simulink model "ZAD2_1_Model"  (R2018a)
settings: Solver=ode45  StartTime=0.0  StopTime=tend  MaxStep=Tp  RelTol=1e-3
values from neighbouring files (symbols this model uses):
  b1 = (eta1^2) *b1 + bm1 + (km1*kb1)/R1    (= 0.00702436843727)    [ZAD0_SRManCw3_Init.m]
  b2 = (eta2^2) *b2 + bm2 + (km2*kb2)/R2    (= 0.00687174794339)    [ZAD0_SRManCw3_Init.m]
  eta = diag([eta1; eta2])    [ZAD0_SRManCw3_Init.m]
  initConditionsPos = [-pi/2; 0]    [ZAD0_SRManCw3_Init.m]
  initConditionsVel = [0; 0]    [ZAD0_SRManCw3_Init.m]
  invR = inv(R)    [ZAD0_SRManCw3_Init.m]
  J1 = Jm1 + (eta1^2) * Jl1    (= 0.000358828993824)    [ZAD0_SRManCw3_Init.m]
  J2 = Jm2 + eta2^2*Jl2    (= 0.000193490125454)    [ZAD0_SRManCw3_Init.m]
  kc1 = 1 / sqrt(kd1 / ki1)    [ZAD0_SRManCw3_Init.m]
  kc2 = 1 / sqrt(kd2 / ki2)    [ZAD0_SRManCw3_Init.m]
  kd1 = omega_n1*zeta1*(2 + lambda1)*J1 - b1    (= 0.0101994232663)    [ZAD0_SRManCw3_Init.m]
  kd2 = omega_n2*zeta2*(2 + lambda2)*J2 - b2    (= 9.38965729567e-05)    [ZAD0_SRManCw3_Init.m]
  ki1 = (omega_n1^3) *lambda1*zeta1*J1    (= 0.465042375996)    [ZAD0_SRManCw3_Init.m]
  ki2 = (omega_n2^3) * lambda2*zeta2*J2    (= 0.167175468392)    [ZAD0_SRManCw3_Init.m]
  Km = diag([km1; km2])    [ZAD0_SRManCw3_Init.m]
  km1 = km    (= 0.0782)    [ZAD0_SRManCw3_Init.m]
  km2 = km    (= 0.0782)    [ZAD0_SRManCw3_Init.m]
  kp1 = (omega_n1^2) * (1 + 2*lambda1*zeta1^2)*J1    (= 0.16793196911)    [ZAD0_SRManCw3_Init.m]
  kp2 = (omega_n2^2) *(1 + 2*lambda2*zeta2^2)*J2    (= 0.0626908006471)    [ZAD0_SRManCw3_Init.m]
  omega1 = 0.6    [ZAD0_SRManCw3_Init.m]
  omega2 = 0.7    [ZAD0_SRManCw3_Init.m]
  Qd01 = 0.65    [ZAD0_SRManCw3_Init.m]
  Qd02 = 0.65    [ZAD0_SRManCw3_Init.m]
  Qd1 = 1.2    [ZAD0_SRManCw3_Init.m]
  Qd11 = 0.75    [ZAD0_SRManCw3_Init.m]
  Qd12 = 0.78    [ZAD0_SRManCw3_Init.m]
  Qd1const = 0.7    [ZAD0_SRManCw3_Init.m]
  Qd2 = 1.3    [ZAD0_SRManCw3_Init.m]
  Qd21 = 0.70    (= 0.7)    [ZAD0_SRManCw3_Init.m]
  Qd22 = 0.98    [ZAD0_SRManCw3_Init.m]
  Qd2const = 0.8    [ZAD0_SRManCw3_Init.m]
  Qd31 = 0.45    [ZAD0_SRManCw3_Init.m]
  Qd32 = 0.90    (= 0.9)    [ZAD0_SRManCw3_Init.m]
  R1 = R    (= 0.917)    [ZAD0_SRManCw3_Init.m]
  R2 = R    (= 0.917)    [ZAD0_SRManCw3_Init.m]
libraries: simulink x2
settings Model: Creator=szymon  LastModifiedBy=szymon

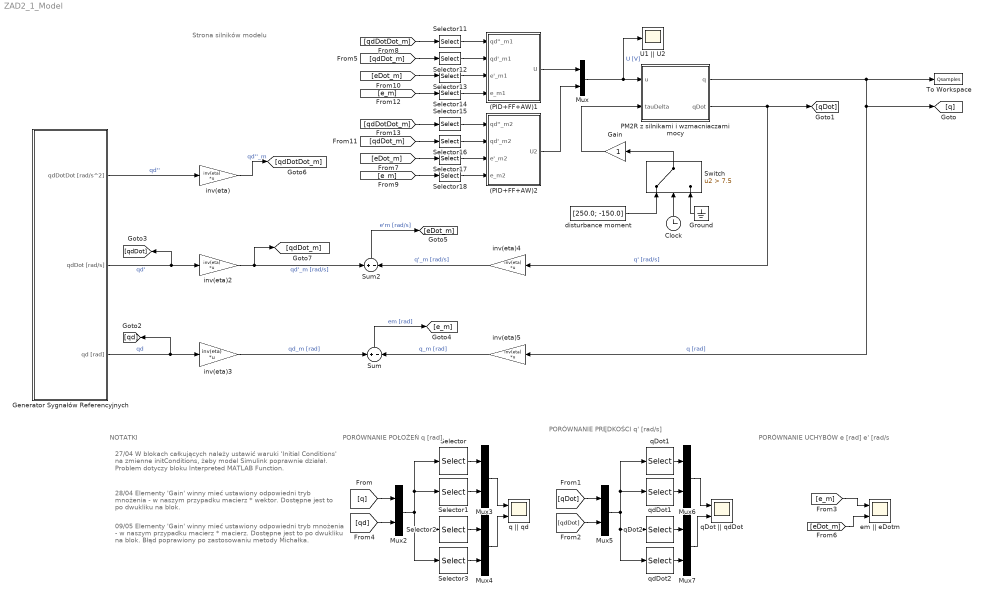
== system ZAD2_1_Model ==
  note: Strona silników modelu
  note: PORÓWNANIE POŁOŻEŃ
      | q [rad]
  note: NOTATKI
  note: 27/04 W blokach całkujących należy ustawić waruki
      | 'Initial Conditions' na zmienne initConditions, żeby model
      | Simulink poprawnie działał. Problem dotyczy bloku
      | Interpreted MATLAB Function.
  note: 28/04 Elementy 'Gain' winny mieć ustawiony odpowiedni tryb
      | mnożenia - w naszym przypadku macierz * wektor.
      | Dostępne jest to po dwukliku na blok.
  note: PORÓWNANIE PRĘDKOŚCI
      | q' [rad/s]
  note: 09/05 Elementy 'Gain' winny mieć ustawiony odpowiedni tryb
      | mnożenia - w naszym przypadku macierz * macierz.
      | Dostępne jest to po dwukliku na blok. Błąd poprawiony po
      | zastosowaniu metody Michałka.
  note: PORÓWNANIE UCHYBÓW
      | e  [rad]
      | e' [rad/s
  (PID+FF+AW)1 : Subsystem
  (PID+FF+AW)2 : Subsystem
  Clock : Clock
  Gain : Gain
  Generator Sygnałów Referencyjnych : Subsystem
  Ground : Ground
  Mux{,2..7} (7 alike) : Mux  Inputs=2
  PM2R z silnikami i wzmacniaczami mocy : Subsystem
  Selector : Selector  InputPortWidth=4  IndexOptions=Index vector (dialog)  Indices=[1]  OutputSizes=1
  Selector1 : Selector  InputPortWidth=4  IndexOptions=Index vector (dialog)  Indices=[3]  OutputSizes=1
  Selector{11..14} (4 alike) : Selector  InputPortWidth=2  IndexOptions=Index vector (dialog)  Indices=[1]  OutputSizes=1
  Selector{15..18} (4 alike) : Selector  InputPortWidth=2  IndexOptions=Index vector (dialog)  Indices=[2]  OutputSizes=1
  Selector2 : Selector  InputPortWidth=4  IndexOptions=Index vector (dialog)  Indices=[2]  OutputSizes=1
  Selector3 : Selector  InputPortWidth=4  IndexOptions=Index vector (dialog)  Indices=[4]  OutputSizes=1
  Sum : Sum  Inputs=+-
  Sum2 : Sum  Inputs=+-
  Switch : Switch  Criteria=u2 > Threshold  Threshold=7.5
  To Workspace : ToWorkspace  VariableName=Qsamples  SampleTime=-1
  U1 || U2 : Scope
  disturbance moment : Constant  Value=[250.0; -150.0]
  em || eDotm : Scope  NumInputPorts=2
  inv(eta){,2..5} (5 alike) : Gain  Gain=inv(eta)  Multiplication=Matrix(K*u)
  q || qd : Scope  NumInputPorts=2
  qDot || qdDot : Scope  NumInputPorts=2
  qDot1 : Selector  InputPortWidth=4  IndexOptions=Index vector (dialog)  Indices=[1]  OutputSizes=1
  qDot2 : Selector  InputPortWidth=4  IndexOptions=Index vector (dialog)  Indices=[2]  OutputSizes=1
  qdDot1 : Selector  InputPortWidth=4  IndexOptions=Index vector (dialog)  Indices=[3]  OutputSizes=1
  qdDot2 : Selector  InputPortWidth=4  IndexOptions=Index vector (dialog)  Indices=[4]  OutputSizes=1
  wires:
  PM2R z silnikami i wzmacniaczami mocy/2(qDot) -> inv(eta)4/1, [qDot]  "q' [rad/s]"
  PM2R z silnikami i wzmacniaczami mocy/1(q) -> inv(eta)5/1, [q], To Workspace/1  "q [rad]"
  [q] -> Mux2/1
  [qd] -> Mux2/2
  Selector/1 -> Mux3/1
  Selector1/1 -> Mux3/2
  Selector2/1 -> Mux4/1
  Selector3/1 -> Mux4/2
  Mux2/1 -> Selector3/1, Selector2/1, Selector1/1, Selector/1
  Mux3/1 -> q || qd/1
  Mux4/1 -> q || qd/2
  qDot2/1 -> Mux7/1
  Mux6/1 -> qDot || qdDot/1
  Mux7/1 -> qDot || qdDot/2
  qdDot2/1 -> Mux7/2
  [qDot] -> Mux5/1
  qdDot1/1 -> Mux6/2
  [qdDot] -> Mux5/2
  qDot1/1 -> Mux6/1
  Mux5/1 -> qdDot2/1, qDot2/1, qdDot1/1, qDot1/1
  Generator Sygnałów Referencyjnych/2(qdDot [rad/s]) -> [qdDot], inv(eta)2/1  "qd'"
  Generator Sygnałów Referencyjnych/1(qdDotDot [rad/s^2]) -> inv(eta)/1  "qd''"
  inv(eta)2/1 -> [qdDot_m], Sum2/1  "qd'_m [rad/s]"
  Mux/1 -> U1 || U2/1, PM2R z silnikami i wzmacniaczami mocy/1(u)  "U [V]"
  Sum2/1 -> [eDot_m]  "e'm [rad/s]"
  Sum/1 -> [e_m]  "em [rad]"
  Selector11/1 -> (PID+FF+AW)1/1(qd''_m1)
  Selector12/1 -> (PID+FF+AW)1/2(qd'_m1)
  Selector13/1 -> (PID+FF+AW)1/3(e'_m1)
  Selector14/1 -> (PID+FF+AW)1/4(e_m1)
  Selector15/1 -> (PID+FF+AW)2/1(qd''_m2)
  Selector16/1 -> (PID+FF+AW)2/2(qd'_m2)
  Selector17/1 -> (PID+FF+AW)2/3(e'_m2)
  Selector18/1 -> (PID+FF+AW)2/4(e_m2)
  (PID+FF+AW)1/1(U) -> Mux/1
  [e_m] -> em || eDotm/1
  inv(eta)4/1 -> Sum2/2  "q'_m [rad/s]"
  inv(eta)5/1 -> Sum/2  "q_m [rad]"
  (PID+FF+AW)2/1(U2) -> Mux/2
  [qdDot_m] -> Selector12/1
  inv(eta)/1 -> [qdDotDot_m]  "qd''_m"
  [qdDotDot_m] -> Selector11/1
  [eDot_m] -> Selector13/1
  [e_m] -> Selector14/1
  [eDot_m] -> Selector17/1
  [qdDot_m] -> Selector16/1
  [e_m] -> Selector18/1
  [qdDotDot_m] -> Selector15/1
  inv(eta)3/1 -> Sum/1  "qd_m [rad]"
  Generator Sygnałów Referencyjnych/3(qd [rad]) -> [qd], inv(eta)3/1  "qd"
  [eDot_m] -> em || eDotm/2
  Switch/1 -> Gain/1
  Ground/1 -> Switch/3
  Clock/1 -> Switch/2
  disturbance moment/1 -> Switch/1
  Gain/1 -> PM2R z silnikami i wzmacniaczami mocy/2(tauDelta)

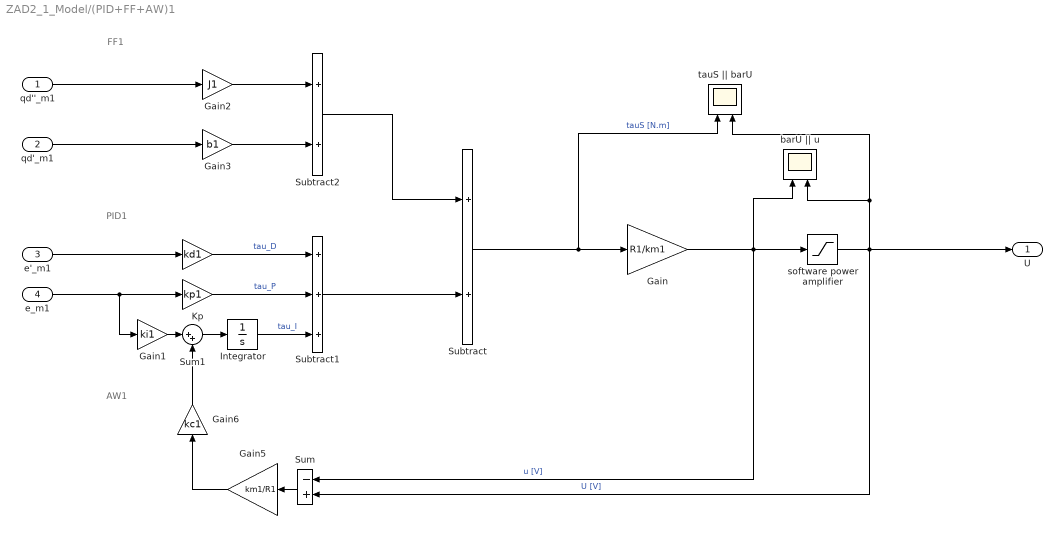
== system ZAD2_1_Model/(PID+FF+AW)1 ==
  note: AW1
  note: FF1
  note: PID1
  qd''_m1 : Inport
  qd'_m1 : Inport  Port=2
  e'_m1 : Inport  Port=3
  e_m1 : Inport  Port=4
  " " : Gain  Gain=kd1
  Gain : Gain  Gain=R1/km1
  Gain1 : Gain  Gain=ki1
  Gain2 : Gain  Gain=J1
  Gain3 : Gain  Gain=b1
  Gain5 : Gain  Gain=km1/R1
  Gain6 : Gain  Gain=kc1
  Integrator : Integrator
  Kp : Gain  Gain=kp1
  Subtract : Sum
  Subtract1 : Sum  Inputs=+++
  Subtract2 : Sum
  Sum : Sum  Inputs=-+
  Sum1 : Sum  Inputs=|++
  barU || u : Scope  NumInputPorts=2
  software power amplifier : Saturate  UpperLimit=24.0  LowerLimit=-24.0
  tauS || barU : Scope  NumInputPorts=2
  U : Outport
  wires:
  Subtract1/1 -> Subtract/2
  Subtract2/1 -> Subtract/1
  Subtract/1 -> Gain/1, tauS || barU/1  "tauS [N.m]"
  software power amplifier/1 -> U/1, tauS || barU/2, barU || u/2, Sum/2  "U [V]"
  e'_m1/1 -> " "/1
  " "/1 -> Subtract1/1  "tau_D"
  Kp/1 -> Subtract1/2  "tau_P"
  qd'_m1/1 -> Gain3/1
  Gain3/1 -> Subtract2/2
  Gain2/1 -> Subtract2/1
  qd''_m1/1 -> Gain2/1
  Gain6/1 -> Sum1/2
  Gain/1 -> Sum/1, software power amplifier/1, barU || u/1  "u [V]"
  Sum/1 -> Gain5/1
  Gain5/1 -> Gain6/1
  e_m1/1 -> Gain1/1, Kp/1
  Integrator/1 -> Subtract1/3  "tau_I"
  Gain1/1 -> Sum1/1
  Sum1/1 -> Integrator/1

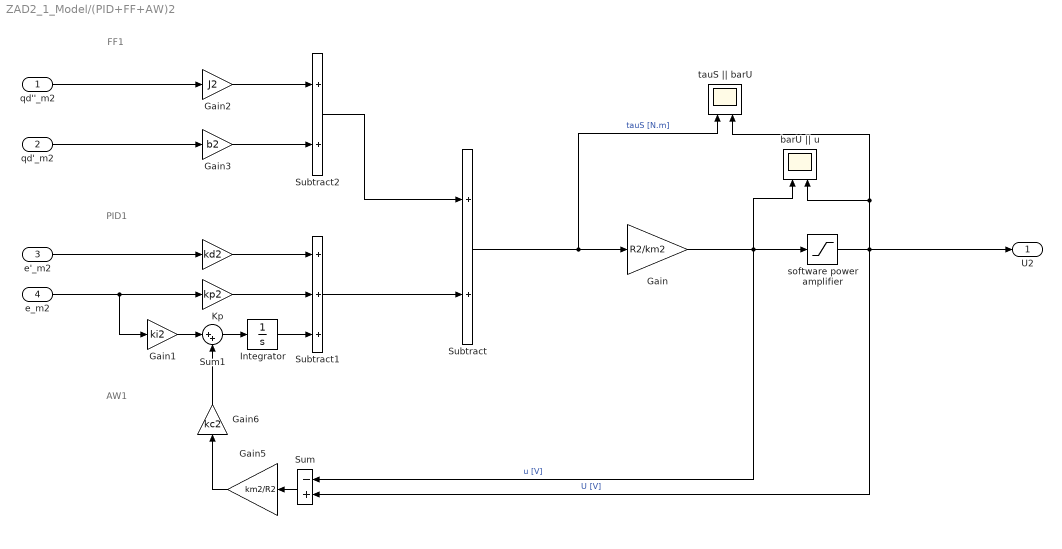
== system ZAD2_1_Model/(PID+FF+AW)2 ==
  note: PID1
  note: FF1
  note: AW1
  qd''_m2 : Inport
  qd'_m2 : Inport  Port=2
  e'_m2 : Inport  Port=3
  e_m2 : Inport  Port=4
  " " : Gain  Gain=kd2
  Gain : Gain  Gain=R2/km2
  Gain1 : Gain  Gain=ki2
  Gain2 : Gain  Gain=J2
  Gain3 : Gain  Gain=b2
  Gain5 : Gain  Gain=km2/R2
  Gain6 : Gain  Gain=kc2
  Integrator : Integrator
  Kp : Gain  Gain=kp2
  Subtract : Sum
  Subtract1 : Sum  Inputs=+++
  Subtract2 : Sum
  Sum : Sum  Inputs=-+
  Sum1 : Sum  Inputs=|++
  barU || u : Scope  NumInputPorts=2
  software power amplifier : Saturate  UpperLimit=24.0  LowerLimit=-24.0
  tauS || barU : Scope  NumInputPorts=2
  U2 : Outport
  wires:
  Gain6/1 -> Sum1/2
  e'_m2/1 -> " "/1
  Subtract1/1 -> Subtract/2
  software power amplifier/1 -> U2/1, tauS || barU/2, barU || u/2, Sum/2  "U [V]"
  Integrator/1 -> Subtract1/3
  qd'_m2/1 -> Gain3/1
  qd''_m2/1 -> Gain2/1
  Subtract2/1 -> Subtract/1
  Gain3/1 -> Subtract2/2
  Gain2/1 -> Subtract2/1
  Sum1/1 -> Integrator/1
  Gain1/1 -> Sum1/1
  " "/1 -> Subtract1/1
  Sum/1 -> Gain5/1
  Gain5/1 -> Gain6/1
  Kp/1 -> Subtract1/2
  e_m2/1 -> Gain1/1, Kp/1
  Gain/1 -> Sum/1, software power amplifier/1, barU || u/1  "u [V]"
  Subtract/1 -> Gain/1, tauS || barU/1  "tauS [N.m]"

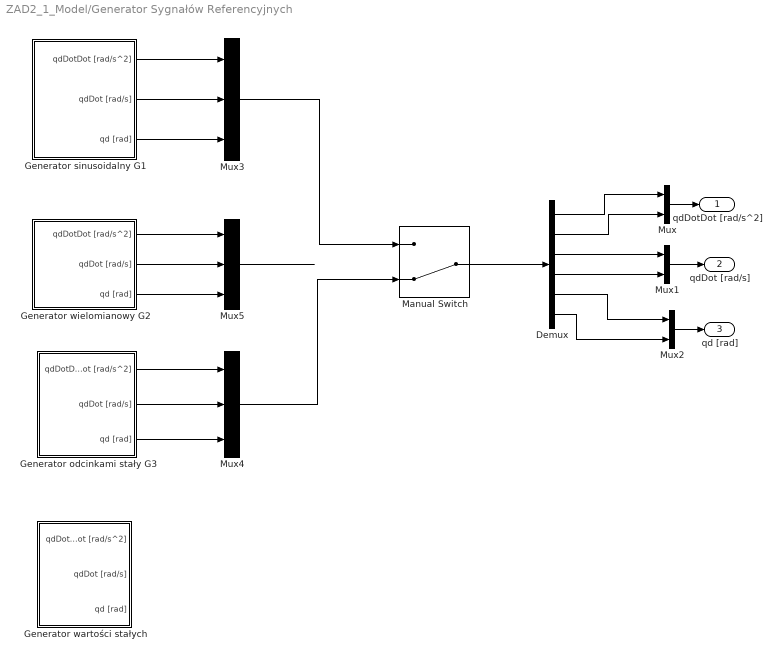
== system ZAD2_1_Model/Generator Sygnałów Referencyjnych ==
  Demux : Demux  Outputs=6
  "Generator odcinkami stały G3 " : Subsystem
  Generator sinusoidalny G1 : Subsystem
  Generator wielomianowy G2 : Subsystem
  Generator wartości stałych : Subsystem
  Manual Switch : ManualSwitch  CurrentSetting=0
  Mux : Mux  Inputs=2
  Mux1 : Mux  Inputs=2
  Mux2 : Mux  Inputs=2
  Mux3 : Mux  Inputs=3
  Mux4 : Mux  Inputs=3
  Mux5 : Mux  Inputs=3
  qdDotDot [rad/s^2] : Outport
  qdDot [rad/s] : Outport  Port=2
  qd [rad] : Outport  Port=3
  wires:
  Mux/1 -> qdDotDot [rad/s^2]/1
  Mux2/1 -> qd [rad]/1
  Mux1/1 -> qdDot [rad/s]/1
  Manual Switch/1 -> Demux/1
  Demux/1 -> Mux/1
  Demux/2 -> Mux/2
  Demux/3 -> Mux1/1
  Demux/4 -> Mux1/2
  Demux/5 -> Mux2/1
  Demux/6 -> Mux2/2
  Generator sinusoidalny G1/2(qdDot [rad/s]) -> Mux3/2
  Generator sinusoidalny G1/1(qdDotDot [rad/s^2]) -> Mux3/1
  Generator sinusoidalny G1/3(qd [rad]) -> Mux3/3
  Mux3/1 -> Manual Switch/1
  "Generator odcinkami stały G3 "/1(qdDotDot [rad/s^2]) -> Mux4/1
  "Generator odcinkami stały G3 "/2(qdDot [rad/s]) -> Mux4/2
  "Generator odcinkami stały G3 "/3(qd [rad]) -> Mux4/3
  Mux4/1 -> Manual Switch/2
  Generator wielomianowy G2/1(qdDotDot [rad/s^2]) -> Mux5/1
  Generator wielomianowy G2/2(qdDot [rad/s]) -> Mux5/2
  Generator wielomianowy G2/3(qd [rad]) -> Mux5/3
  Mux5/1 -> ?

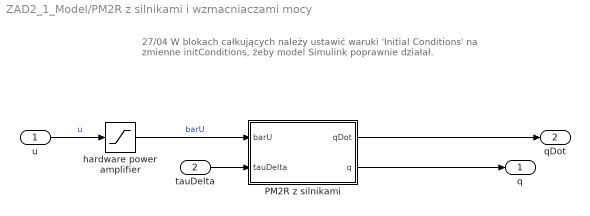
== system ZAD2_1_Model/PM2R z silnikami i wzmacniaczami mocy ==
  note: 27/04 W blokach całkujących należy ustawić waruki 'Initial Conditions' na
      | zmienne initConditions, żeby model Simulink poprawnie działał.
  u : Inport
  tauDelta : Inport  Port=2
  PM2R z silnikami : Subsystem
  hardware power amplifier : Saturate  UpperLimit=24.0  LowerLimit=-24.0
  q : Outport
  qDot : Outport  Port=2
  wires:
  u/1 -> hardware power amplifier/1  "u"
  PM2R z silnikami/1(qDot) -> qDot/1
  PM2R z silnikami/2(q) -> q/1
  tauDelta/1 -> PM2R z silnikami/2(tauDelta)
  hardware power amplifier/1 -> PM2R z silnikami/1(barU)  "barU"

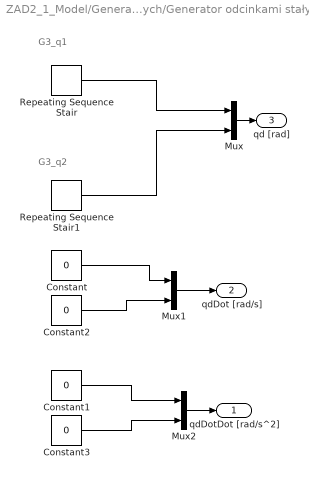
== system ZAD2_1_Model/Generator Sygnałów Referencyjnych/Generator odcinkami stały G3  ==
  note: G3_q2
  note: G3_q1
  Constant{,1..3} (4 alike) : Constant  Value=0
  Mux : Mux  Inputs=2
  Mux1 : Mux  Inputs=2
  Mux2 : Mux  Inputs=2
  Repeating Sequence Stair : simulink/Sources/Repeating Sequence Stair  OutValues=[Qd1const 0].'  tsamp=Ta  OutMin=[]  OutMax=[]  OutDataTypeStr=double  OutputDataTypeScalingMode=double  OutDataType=fixdt(0,8)  ConRadixGroup=Best Precision: Vector-wise  OutScaling=2^-12
  Repeating Sequence Stair1 : simulink/Sources/Repeating Sequence Stair  OutValues=[Qd2const 0].'  tsamp=Tb  OutMin=[]  OutMax=[]  OutDataTypeStr=double  OutputDataTypeScalingMode=double  OutDataType=fixdt(0,8)  ConRadixGroup=Best Precision: Vector-wise  OutScaling=2^-12
  qdDotDot [rad/s^2] : Outport
  qdDot [rad/s] : Outport  Port=2
  qd [rad] : Outport  Port=3
  wires:
  Constant/1 -> Mux1/1
  Repeating Sequence Stair1/1 -> Mux/2
  Repeating Sequence Stair/1 -> Mux/1
  Mux/1 -> qd [rad]/1
  Constant1/1 -> Mux2/1
  Constant2/1 -> Mux1/2
  Constant3/1 -> Mux2/2
  Mux2/1 -> qdDotDot [rad/s^2]/1
  Mux1/1 -> qdDot [rad/s]/1

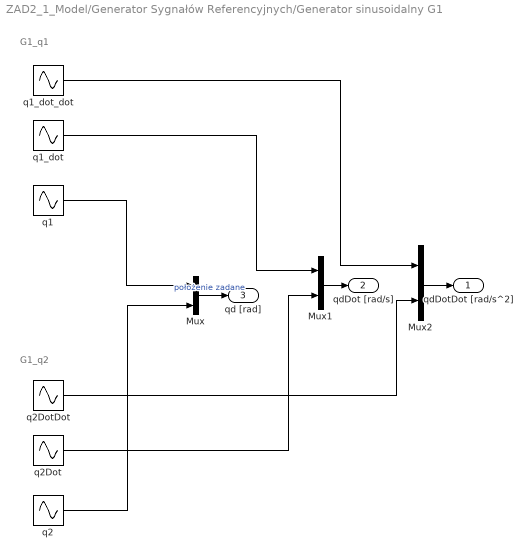
== system ZAD2_1_Model/Generator Sygnałów Referencyjnych/Generator sinusoidalny G1 ==
  note: G1_q1
  note: G1_q2
  Mux : Mux  Inputs=2
  Mux1 : Mux  Inputs=2
  Mux2 : Mux  Inputs=2
  "q1 " : Sin  Amplitude=Qd1  Frequency=omega1  SampleTime=0
  q1_dot : Sin  Amplitude=omega1*Qd1  Frequency=omega1  Phase=pi/2  SampleTime=0
  "q1_dot_dot " : Sin  Amplitude=-omega1^2*Qd1  Frequency=omega1  SampleTime=0
  q2 : Sin  Amplitude=Qd2  Frequency=omega2  SampleTime=0
  q2Dot : Sin  Amplitude=omega2*Qd2  Frequency=omega2  Phase=pi/2  SampleTime=0
  "q2DotDot " : Sin  Amplitude=-omega2^2*Qd2  Frequency=omega2  SampleTime=0
  qdDotDot [rad/s^2] : Outport
  qdDot [rad/s] : Outport  Port=2
  qd [rad] : Outport  Port=3
  wires:
  Mux1/1 -> qdDot [rad/s]/1
  Mux2/1 -> qdDotDot [rad/s^2]/1
  "q1_dot_dot "/1 -> Mux2/1
  "q2DotDot "/1 -> Mux2/2
  q2Dot/1 -> Mux1/2
  q1_dot/1 -> Mux1/1
  q2/1 -> Mux/2
  "q1 "/1 -> Mux/1
  Mux/1 -> qd [rad]/1  "położenie zadane"

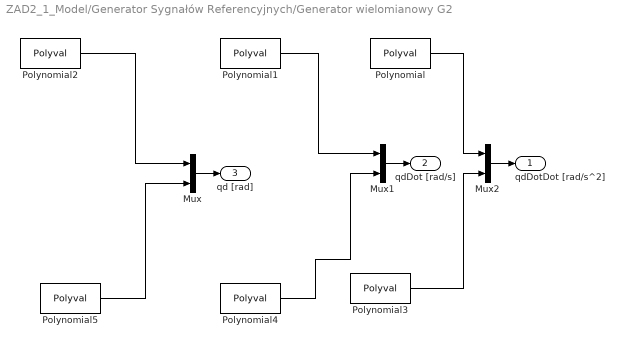
== system ZAD2_1_Model/Generator Sygnałów Referencyjnych/Generator wielomianowy G2 ==
  Mux : Mux  Inputs=2
  Mux1 : Mux  Inputs=2
  Mux2 : Mux  Inputs=2
  Polynomial : Polyval  Coefs=[6*Qd31*t, 2*Qd21]
  Polynomial1 : Polyval  Coefs=[3*Qd31*t.^2, 2*Qd21*t, Qd11]
  Polynomial2 : Polyval  Coefs=[Qd31*t.^3, Qd21*t.^2, Qd11*t, Qd01]
  Polynomial3 : Polyval  Coefs=[6*Qd32*t, 2*Qd22]
  Polynomial4 : Polyval  Coefs=[3*Qd32*t.^2, 2*Qd22*t, Qd12]
  Polynomial5 : Polyval  Coefs=[Qd32*t.^3, Qd22*t.^2, Qd12*t, Qd02]
  qdDotDot [rad/s^2] : Outport
  qdDot [rad/s] : Outport  Port=2
  qd [rad] : Outport  Port=3
  wires:
  Polynomial/1 -> Mux2/1
  Polynomial1/1 -> Mux1/1
  Polynomial2/1 -> Mux/1
  Polynomial3/1 -> Mux2/2
  Polynomial5/1 -> Mux/2
  Polynomial4/1 -> Mux1/2
  Mux/1 -> qd [rad]/1
  Mux1/1 -> qdDot [rad/s]/1
  Mux2/1 -> qdDotDot [rad/s^2]/1

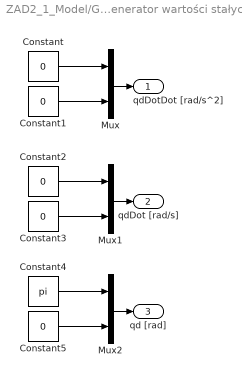
== system ZAD2_1_Model/Generator Sygnałów Referencyjnych/Generator wartości stałych ==
  Constant{,1..3,5} (5 alike) : Constant  Value=0
  Constant4 : Constant  Value=pi
  Mux : Mux  Inputs=2
  Mux1 : Mux  Inputs=2
  Mux2 : Mux  Inputs=2
  qdDotDot [rad/s^2] : Outport
  qdDot [rad/s] : Outport  Port=2
  qd [rad] : Outport  Port=3
  wires:
  Constant/1 -> Mux/1
  Mux/1 -> qdDotDot [rad/s^2]/1
  Constant1/1 -> Mux/2
  Constant2/1 -> Mux1/1
  Constant3/1 -> Mux1/2
  Mux1/1 -> qdDot [rad/s]/1
  Constant4/1 -> Mux2/1
  Constant5/1 -> Mux2/2
  Mux2/1 -> qd [rad]/1

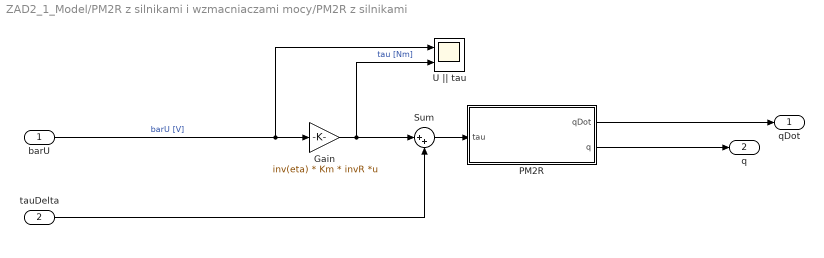
== system ZAD2_1_Model/PM2R z silnikami i wzmacniaczami mocy/PM2R z silnikami ==
  barU : Inport
  tauDelta : Inport  Port=2
  Gain : Gain  Gain=inv(eta) * Km * invR  Multiplication=Matrix(K*u)
  PM2R : Subsystem
  Sum : Sum  Inputs=|++
  U || tau : Scope  NumInputPorts=2
  qDot : Outport
  q : Outport  Port=2
  wires:
  Gain/1 -> Sum/1, U || tau/2  "tau [Nm]"
  PM2R/2(q) -> q/1
  PM2R/1(qDot) -> qDot/1
  barU/1 -> U || tau/1, Gain/1  "barU [V]"
  Sum/1 -> PM2R/1(tau)
  tauDelta/1 -> Sum/2

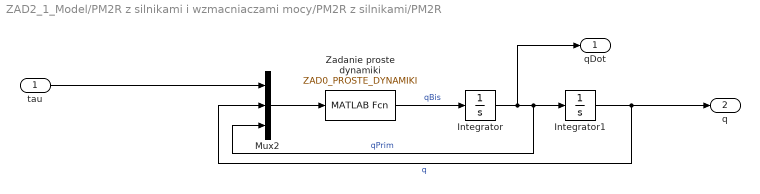
== system ZAD2_1_Model/PM2R z silnikami i wzmacniaczami mocy/PM2R z silnikami/PM2R ==
  tau : Inport
  Integrator : Integrator  InitialCondition=initConditionsVel
  Integrator1 : Integrator  InitialCondition=initConditionsPos
  Mux2 : Mux  Inputs=3
  Zadanie proste dynamiki : MATLABFcn  MATLABFcn=ZAD0_PROSTE_DYNAMIKI
  qDot : Outport
  q : Outport  Port=2
  wires:
  Mux2/1 -> Zadanie proste dynamiki/1
  Integrator1/1 -> q/1, Mux2/2  "q"
  Integrator/1 -> qDot/1, Mux2/3, Integrator1/1  "qPrim"
  Zadanie proste dynamiki/1 -> Integrator/1  "qBis"
  tau/1 -> Mux2/1
